simulink model "boost_and_two_level__1_sm_controller"  (R2021b)
settings: Solver=ode3  StartTime=0.0  StopTime=inf  FixedStep=2e-05  RelTol=1e-3
PostLoadFcn:
  | Boost_and_Two_Level_Inverter_param;
InitFcn:
  | Boost_and_Two_Level_Inverter_param;
undefined symbols (not defined in the file or in its folder): af15, arm1_g1, Boost2lvl_SFun, boost_I, boost_V, c62c8459, eHSx128_Gen4_Machines_IOConfig1, EX, fault_sw, Inv_PWM_Phases, Ts, v1, VC707_2, vin, vsrc1, vsrc2, vsrc3
libraries: opal_lib x5, rtio_opalrt_common x2, rtlab x1, ehsSchematicEditorSourceLib x1
PreSaveFcn:
  | try, efsUpdateVersionAnnotation, end
settings Model: ARTEMISmethode_block_infos=$$__separator__$$  Creator=PYRobert  LastModifiedBy=Grogu
settings SolverCC: AlgebraicLoopSolver=TrustRegion
settings DataIOCC: LimitDataPoints=on  SaveFormat=Array  SignalLoggingSaveFormat=ModelDataLogs  SaveOutput=off  SignalLogging=off  SaveTime=off  ReturnWorkspaceOutputs=off  SignalLoggingName=sigsOut
settings OptimizationCC: BlockReduction=off  OptimizeBlockIOStorage=off  BufferReuse=off  GlobalBufferReuse=off  ExpressionFolding=off  ExpressionDepthLimit=2147483647  LocalBlockOutputs=off  InitFltsAndDblsToZero=on  LifeSpan=inf  OptimizeDataStoreBuffers=off  BusAssignmentInplaceUpdate=off
settings DebuggingCC: SaveWithParameterizedLinksMsg=none  UnderspecifiedInitializationDetection=Classic  MergeDetectMultiDrivingBlocksExec=none  SignalResolutionControl=TryResolveAllWithWarning  InheritedTsInSrcMsg=none  MultiTaskDSMMsg=warning  MultiTaskCondExecSysMsg=none  ParameterOverflowMsg=none  FcnCallInpInsideContextMsg=warning  StateNameClashWarn=warning  SFUnexpectedBacktrackingDiag=warning  SFNoUnconditionalDefaultTransitionDiag=warning  SFExecutionAtInitializationDiag=none  SFMachineParentedDataDiag=warning  ArithmeticOperatorsInVariantConditions=warning
settings HardwareCC: ProdBitPerLong=64  ProdHWDeviceType=Intel->x86-64 (Linux 64)  TargetBitPerPointer=64  TargetBitPerSizeT=64  TargetBitPerPtrDiffT=64  TargetLongLongMode=on  TargetIntDivRoundTo=Zero  TargetEndianess=LittleEndian  TargetWordSize=64  TargetHWDeviceType=MATLAB Host  ProdEqTarget=off
settings ModelReferenceCC: PropagateSignalLabelsOutOfModel=off
settings SFSimCC: SimUseLocalCustomCode=off  CustomCodeUndefinedFunction=UseInterfaceOnly
settings RTWCC: GenCodeOnly=on  RTWUseLocalCustomCode=off
settings CodeAppCC: StateflowObjectComments=on
settings GRTTargetCC: TargetFcnLib=ansi_tfl_tmw.mat  TargetLangStandard=C89/C90 (ANSI)  CombineOutputUpdateFcns=off  GRTInterface=on
settings ConfigComp: CovMetricSettings=dw  CovSaveCumulativeToWorkspaceVar=on  CovSaveSingleToWorkspaceVar=on  CovExternalEMLEnable=off  CovSFcnEnable=off
settings SimscapeCC: SimscapeNormalizeSystem=off

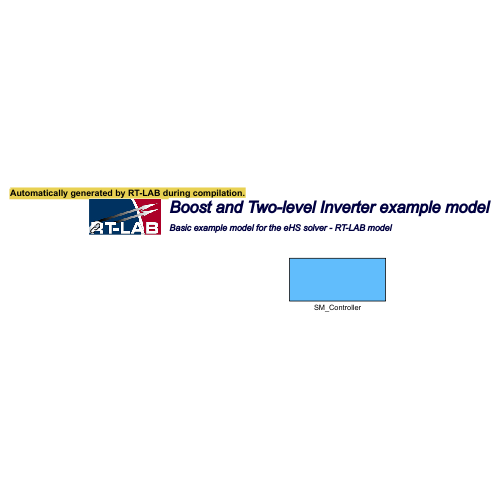
[thumbnail: Simulink's stored preview of the top-level diagram]
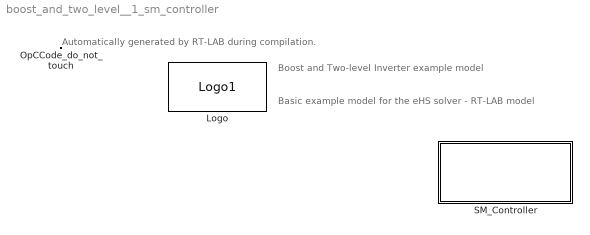
== system boost_and_two_level__1_sm_controller ==
  note: Boost and Two-level Inverter example model
  note: Basic example model for the eHS solver - RT-LAB model
  note: Automatically generated by RT-LAB during compilation.
  Logo : opal_lib/Logo1  vide=[]
  OpCCode_do_not_touch : opal_lib/Communication/OpCCode  SystemSampleTime=-1  VariantActivationTime=update diagram  Latency=0  AutoFrameSizeCalculation=off
  SM_Controller : Subsystem

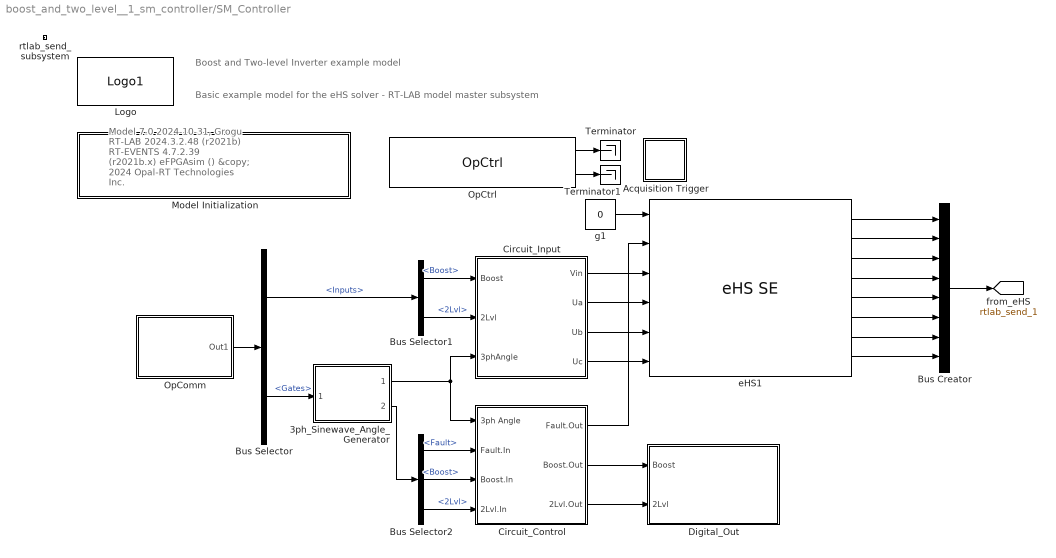
== system boost_and_two_level__1_sm_controller/SM_Controller ==
  note: Model 7.0 2024-10-31, Grogu
      | RT-LAB 2024.3.2.48 (r2021b)
      | RT-EVENTS 4.7.2.39 (r2021b.x)
      | eFPGAsim ()
      | &copy; 2024 Opal-RT Technologies Inc.
  note: Boost and Two-level Inverter example model
  note: Basic example model for the eHS solver - RT-LAB model master subsystem
  3ph_Sinewave_Angle_Generator : Subsystem
  Acquisition Trigger : Subsystem
  Bus Creator : BusCreator  Inputs=8
  Bus Selector : BusSelector  OutputSignals=Inputs,Gates
  Bus Selector1 : BusSelector  OutputSignals=Boost,2Lvl
  Bus Selector2 : BusSelector  OutputSignals=Fault,Boost,2Lvl
  Circuit_Control : Subsystem
  Circuit_Input : Subsystem
  Digital_Out : Subsystem
  Logo : opal_lib/Logo1  vide=[]
  Model Initialization : Subsystem  mask(Model Functions){InitFcnX=Boost_and_Two_Level_Inverter_param;, prel=off, posl=on, inif=on, strf=off}
      mask prompts: InitFcnX "Initialisation"; prel "Preload Function"; posl "PostLoad Function"; inif "InitFcn"; strf "StartFcn"
      mask init:
      | currentBlock = gcb;
      | root = bdroot(currentBlock);
      | 
      | if ~strcmp(get_param(root,'BlockDiagramType'),'library')
      |     if prel==1
      |         set_param(root, 'PreLoadFcn', InitFcnX);
      |     else
      |         set_param(root, 'PreLoadFcn', '');
      |     end
      |     if inif==1
      |         set_param(root, 'InitFcn', InitFcnX);
      |     else
      |         set_param(root, 'InitFcn', '');
      |     end
      |     if strf==1
      |         set_param(root, 'StartFcn', InitFcnX);
      |     else
      |         set_param(root, 'StartFcn', '');
      |     end
      |     if posl==1
      |         set_param(root, 'PostLoadFcn', InitFcnX);
      |     else
      |         set_param(root, 'PostLoadFcn', '');
      |     end
      | end
      | 
      | pos = get_param(currentBlock, 'Position');
      | width = pos(3) - pos(1); height = pos(4) - pos(2);
      | txt = [ upper(root) '\n' '- InitFcn. . . . . '  get_param(root, 'InitFcn') ];
      settings: CopyFcn=set_param(gcb,'LinkStatus','none')
      mask Display: text(5, height*0.5, txt, 'horizontalAlignment', 'left', 'verticalAlignment', 'middle') ;
  OpComm : Subsystem
      mask init:
      | opmaskdisplay('maskdisplay_block',gcb,'disp(''OpComm'')');
      mask Display:
      | patch([0 0.5 0.7 0],[1 1 0 0],[0.7 0.75 0.9]);
      | patch([1 0.53 0.73 1],[1 1 0 0],[1 0.8 0.7]);
      | plot([0 0 1 1 0],[0 1 1 0 0]);
      | disp('OpComm')
  OpCtrl : rtio_opalrt_common/OpCtrl  CtrlName='OpCtrl'  boardid=0  BitstreamFilename=VC707_2-EX-0001-3_6_0_818-eHSx128_Gen4_Machines_IOConfig1-35-61.bin  numconfig=-1  mode=Master  externalClock=off  decimRtsi=0  calibIO=off  SampleTime=0  loadinport=-1  BoardType=VC707  SecondaryPresent=off  sync_type=Audio  scope_enable=off  fsdFileName=VC707_2-EX-0001-3_4_0_820-eHSx128_Gen4_Machines_IOConfig1-35-4E.fsd  mismatch_disable=off
      settings: SourceProductName=RT-LAB I/O
  Terminator : Terminator
  Terminator1 : Terminator
  eHS1 : ehsSchematicEditorSourceLib/eHS SE  modelName=Boost2lvl_SFun - v1  modelUuid=c62c8459-3f79-48c0-af15-759a73c628dc  modelDisplayName=Boost2lvl_SFun  lastLoadedModelText=Circuit loaded on 09-Oct-2024 14:20:43  lastLoadedModelName=Boost2lvl_SFun - v1  lastLoadedModelUuid=c62c8459-3f79-48c0-af15-759a73c628dc  lastLoadedModelDisplayName=Boost2lvl_SFun - v1  triggerUpdate=on  timeStepInfo=Time Step: 230 ns (Min: 230 ns)  inputPins=arm1_g1,fault_sw,vin,vsrc1,vsrc2,vsrc3  outputPins=2Lvl_Ia,2Lvl_Ib,2Lvl_Ic,2Lvl_Va,2Lvl_Vb,2Lvl_Vc,boost_I,boost_V  loadPassed=1  firmwareName=VC707_2-EX-0001-3_6_0_818-eHSx128_Gen4_Machines_IOConfig1-35-61.bin  driverType=SFUN  ehsEffectiveLicense=x128  migrated=on  opCtrlName='OpCtrl'  autoConfigureFirmware=on  ehsFileName=Boost2lvl_SFun.ehs3  buildReportFile=C:\Working\git-repos\efpgasim-gitlab\efpgasim\Examples\Schematic_Editor_Workflow\eHS_Gen_4\Boost And Two Level Inverter\SFUN\Simulink\models\Boost_and_Two_Level_Inverter_Sfun\EFPGASIMConfig\logs\Boost2lvl_SFun\logs\eHSBuildReport.txt  displayBlockInfos=|
      | x128
      | Time Step: 230 ns (Min: 230 ns)
      settings: AttributesFormatString=%<opCtrlName>\n%<ehsFileName>\n%<displayBlockInfos>
  g1 : Constant  Value=0
  rtlab_send_subsystem : Subsystem  Priority=-100
      mask Display: text(0,0,'');
  tag scope: rtlab_send_1=global
  wires:
  OpComm/1(Out1) -> Bus Selector/1
  Circuit_Control/2(Boost.Out) -> Digital_Out/1(Boost)
  Circuit_Control/3(2Lvl.Out) -> Digital_Out/2(2Lvl)
  Bus Selector1/1 -> Circuit_Input/1(Boost)  "<Boost>"
  Bus Selector1/2 -> Circuit_Input/2(2Lvl)  "<2Lvl>"
  Bus Selector/1 -> Bus Selector1/1  "<Inputs>"
  Bus Selector/2 -> 3ph_Sinewave_Angle_Generator/1(Params.In)  "<Gates>"
  Bus Selector2/3 -> Circuit_Control/4(2Lvl.In)  "<2Lvl>"
  Bus Selector2/2 -> Circuit_Control/3(Boost.In)  "<Boost>"
  Bus Selector2/1 -> Circuit_Control/2(Fault.In)  "<Fault>"
  3ph_Sinewave_Angle_Generator/2(Params.Out) -> Bus Selector2/1
  3ph_Sinewave_Angle_Generator/1(3ph_Angle) -> Circuit_Input/3(3phAngle), Circuit_Control/1(3ph Angle)
  Bus Creator/1 -> [rtlab_send_1]
  Circuit_Control/1(Fault.Out) -> eHS1/2
  Circuit_Input/1(Vin) -> eHS1/3
  Circuit_Input/2(Ua) -> eHS1/4
  Circuit_Input/3(Ub) -> eHS1/5
  Circuit_Input/4(Uc) -> eHS1/6
  eHS1/2 -> Bus Creator/2
  eHS1/3 -> Bus Creator/3
  eHS1/4 -> Bus Creator/4
  eHS1/5 -> Bus Creator/5
  eHS1/6 -> Bus Creator/6
  eHS1/7 -> Bus Creator/7
  eHS1/8 -> Bus Creator/8
  g1/1 -> eHS1/1
  OpCtrl/1 -> Terminator/1
  OpCtrl/2 -> Terminator1/1
  eHS1/1 -> Bus Creator/1

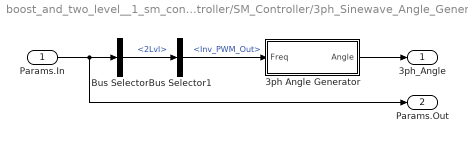
== system boost_and_two_level__1_sm_controller/SM_Controller/3ph_Sinewave_Angle_Generator ==
  Params.In : Inport
  3ph Angle Generator : Subsystem
  Bus Selector : BusSelector  OutputSignals=2Lvl
  Bus Selector1 : BusSelector  OutputSignals=Inv_PWM_Out
  3ph_Angle : Outport  VectorParamsAs1DForOutWhenUnconnected=off
  Params.Out : Outport  Port=2  VectorParamsAs1DForOutWhenUnconnected=off
  wires:
  Params.In/1 -> Params.Out/1, Bus Selector/1
  Bus Selector/1 -> Bus Selector1/1  "<2Lvl>"
  Bus Selector1/1 -> 3ph Angle Generator/1(Freq)  "<Inv_PWM_Out>"
  3ph Angle Generator/1(Angle) -> 3ph_Angle/1

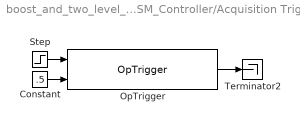
== system boost_and_two_level__1_sm_controller/SM_Controller/Acquisition Trigger ==
  Constant : Constant  Value=.5
  OpTrigger : rtlab/DataLogging/OpTrigger  Trig_Type=TRIGGER SIGNAL >= TRIGGER LEVEL  Trig_Offset=0  Acq_Group=1
      settings: SourceProductName=RT-LAB
  Step : Step  Time=0.5  SampleTime=Ts
  Terminator2 : Terminator
  wires:
  Constant/1 -> OpTrigger/2
  Step/1 -> OpTrigger/1
  OpTrigger/1 -> Terminator2/1

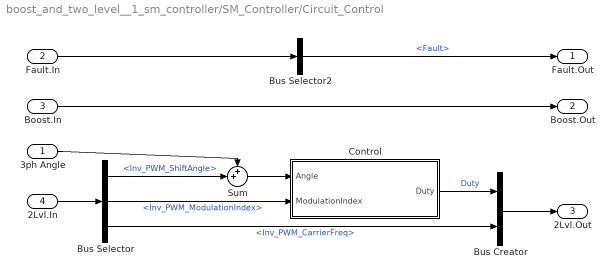
== system boost_and_two_level__1_sm_controller/SM_Controller/Circuit_Control ==
  3ph Angle : Inport
  Fault.In : Inport  Port=2
  Boost.In : Inport  Port=3
  2Lvl.In : Inport  Port=4
  Bus Creator : BusCreator  Inputs=2
  Bus Selector : BusSelector  OutputSignals=Inv_PWM_ShiftAngle,Inv_PWM_ModulationIndex,Inv_PWM_CarrierFreq
  Bus Selector2 : BusSelector  OutputSignals=Fault
  Control : Subsystem
  Sum : Sum  Inputs=++|
  Fault.Out : Outport  VectorParamsAs1DForOutWhenUnconnected=off
  Boost.Out : Outport  Port=2  VectorParamsAs1DForOutWhenUnconnected=off
  2Lvl.Out : Outport  Port=3  VectorParamsAs1DForOutWhenUnconnected=off
  wires:
  Boost.In/1 -> Boost.Out/1
  Bus Creator/1 -> 2Lvl.Out/1
  2Lvl.In/1 -> Bus Selector/1
  Fault.In/1 -> Bus Selector2/1
  Bus Selector2/1 -> Fault.Out/1  "<Fault>"
  Bus Selector/2 -> Control/2(ModulationIndex)  "<Inv_PWM_ModulationIndex>"
  Control/1(Duty) -> Bus Creator/1  "Duty"
  Bus Selector/3 -> Bus Creator/2  "<Inv_PWM_CarrierFreq>"
  Sum/1 -> Control/1(Angle)
  Bus Selector/1 -> Sum/2  "<Inv_PWM_ShiftAngle>"
  3ph Angle/1 -> Sum/1

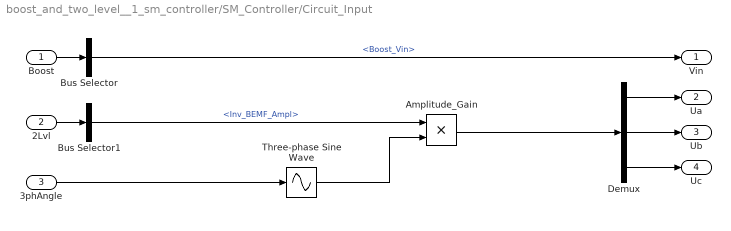
== system boost_and_two_level__1_sm_controller/SM_Controller/Circuit_Input ==
  Boost : Inport
  2Lvl : Inport  Port=2
  3phAngle : Inport  Port=3
  Amplitude_Gain : Product  RndMeth=Zero
  Bus Selector : BusSelector  OutputSignals=Boost_Vin
  Bus Selector1 : BusSelector  OutputSignals=Inv_BEMF_Ampl
  Demux : Demux  Outputs=3
  Three-phase Sine Wave : Sin  TimeSource=Use external signal  Phase=Inv_PWM_Phases
  Vin : Outport  VectorParamsAs1DForOutWhenUnconnected=off
  Ua : Outport  Port=2  VectorParamsAs1DForOutWhenUnconnected=off
  Ub : Outport  Port=3  VectorParamsAs1DForOutWhenUnconnected=off
  Uc : Outport  Port=4  VectorParamsAs1DForOutWhenUnconnected=off
  wires:
  Boost/1 -> Bus Selector/1
  Bus Selector/1 -> Vin/1  "<Boost_Vin>"
  2Lvl/1 -> Bus Selector1/1
  Demux/1 -> Ua/1
  Demux/2 -> Ub/1
  Demux/3 -> Uc/1
  Bus Selector1/1 -> Amplitude_Gain/1  "<Inv_BEMF_Ampl>"
  Amplitude_Gain/1 -> Demux/1
  Three-phase Sine Wave/1 -> Amplitude_Gain/2
  3phAngle/1 -> Three-phase Sine Wave/1

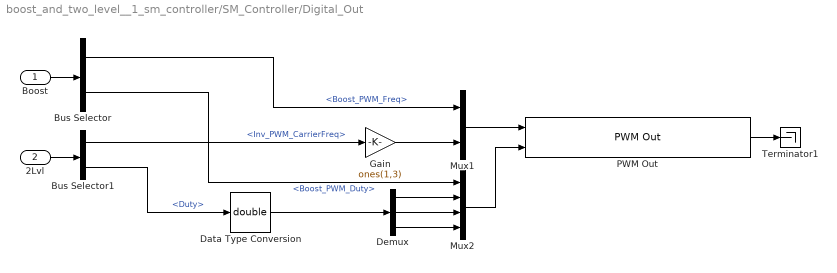
== system boost_and_two_level__1_sm_controller/SM_Controller/Digital_Out ==
  Boost : Inport
  2Lvl : Inport  Port=2
  Bus Selector : BusSelector  OutputSignals=Boost_PWM_Freq,Boost_PWM_Duty
  Bus Selector1 : BusSelector  OutputSignals=Inv_PWM_CarrierFreq,Duty
  Data Type Conversion : DataTypeConversion  OutDataTypeStr=double
  Demux : Demux  Outputs=3
  Gain : Gain  Gain=ones(1,3)
  Mux1 : Mux  Inputs=2
  Mux2 : Mux
  PWM Out : rtio_opalrt_common/PWM Out  CtrlName='OpCtrl'  portNb=11  FcnNos=Slot 2 Module B Subsection 1  size=64  maxcount=8  count=4  polarity=Active High  symMode=Asymmetric  rtPhaseDeadTimeEnabled=on  allowDisablingChannel=off  complementary=off  rtDeadTimeEnabled=off  deadTime=[0 0 0 0]  numchan=4  loadnb=4  rtPhaseShiftEnabled=off  initphase=[0 0 0 0]
      settings: AttributesFormatString=%<CtrlName>  SourceProductName=RT-LAB I/O
  Terminator1 : Terminator
  wires:
  Bus Selector/1 -> Mux1/1  "<Boost_PWM_Freq>"
  Bus Selector/2 -> Mux2/1  "<Boost_PWM_Duty>"
  Boost/1 -> Bus Selector/1
  2Lvl/1 -> Bus Selector1/1
  Bus Selector1/2 -> Data Type Conversion/1  "<Duty>"
  Data Type Conversion/1 -> Demux/1
  Bus Selector1/1 -> Gain/1  "<Inv_PWM_CarrierFreq>"
  Mux1/1 -> PWM Out/1
  Gain/1 -> Mux1/2
  Demux/2 -> Mux2/3
  Demux/1 -> Mux2/2
  Demux/3 -> Mux2/4
  Mux2/1 -> PWM Out/2
  PWM Out/1 -> Terminator1/1

== system boost_and_two_level__1_sm_controller/SM_Controller/Model Initialization ==

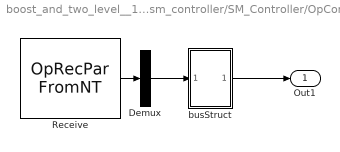
== system boost_and_two_level__1_sm_controller/SM_Controller/OpComm ==
  Demux : Demux  Outputs=[9]
  Receive : opal_lib/Communication/OpRecPar FromNT  Data_width=9  InitialConditions=[100;25;1;10000;0.7;55000;50;0.8;0.00349065850398866]
  busStruct : Subsystem
  Out1 : Outport
  wires:
  Demux/1 -> busStruct/1(In1)
  busStruct/1(Out1) -> Out1/1
  Receive/1 -> Demux/1

== system boost_and_two_level__1_sm_controller/SM_Controller/rtlab_send_subsystem ==
  Subsystem1 : Subsystem
  wires:
  [rtlab_send_1] -> Subsystem1/1(In1)

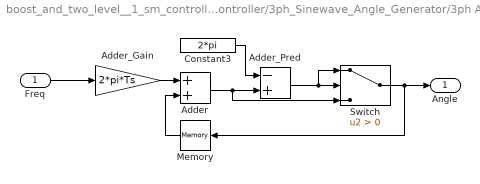
== system boost_and_two_level__1_sm_controller/SM_Controller/3ph_Sinewave_Angle_Generator/3ph Angle Generator ==
  Freq : Inport
  Adder : Sum
  Adder_Gain : Gain  Gain=2*pi*Ts  OutDataTypeStr=double
  Adder_Pred : Sum  Inputs=-+
  Constant3 : Constant  Value=2*pi  OutDataTypeStr=double
  Memory : Memory  InheritSampleTime=on
  Switch : Switch  Criteria=u2 > Threshold
  Angle : Outport  VectorParamsAs1DForOutWhenUnconnected=off
  wires:
  Memory/1 -> Adder/2
  Freq/1 -> Adder_Gain/1
  Adder/1 -> Switch/3, Adder_Pred/2
  Adder_Gain/1 -> Adder/1
  Constant3/1 -> Adder_Pred/1
  Switch/1 -> Angle/1, Memory/1
  Adder_Pred/1 -> Switch/2, Switch/1

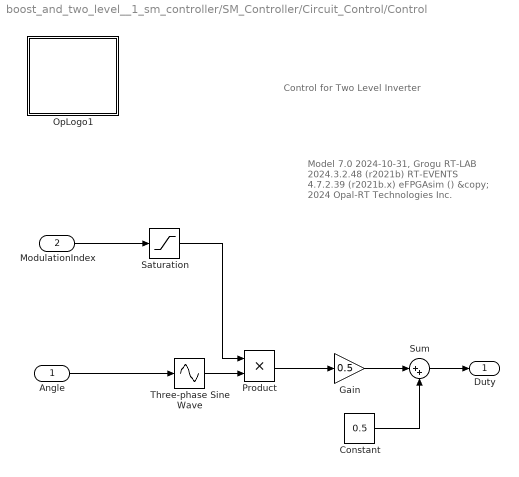
== system boost_and_two_level__1_sm_controller/SM_Controller/Circuit_Control/Control ==
  note: Control for Two Level Inverter
  note: Model 7.0 2024-10-31, Grogu
      | RT-LAB 2024.3.2.48 (r2021b)
      | RT-EVENTS 4.7.2.39 (r2021b.x)
      | eFPGAsim ()
      | &copy; 2024 Opal-RT Technologies Inc.
  Angle : Inport
  ModulationIndex : Inport  Port=2
  Constant : Constant  Value=0.5
  Gain : Gain  Gain=0.5
  OpLogo1 : Subsystem
  Product : Product  RndMeth=Zero
  Saturation : Saturate  UpperLimit=0.95  LowerLimit=0.05  OutDataTypeStr=Inherit: Inherit via back propagation
  Sum : Sum  Inputs=|++
  Three-phase Sine Wave : Sin  TimeSource=Use external signal  Phase=Inv_PWM_Phases
  Duty : Outport  VectorParamsAs1DForOutWhenUnconnected=off
  wires:
  ModulationIndex/1 -> Saturation/1
  Saturation/1 -> Product/1
  Product/1 -> Gain/1
  Gain/1 -> Sum/1
  Sum/1 -> Duty/1
  Constant/1 -> Sum/2
  Angle/1 -> Three-phase Sine Wave/1
  Three-phase Sine Wave/1 -> Product/2

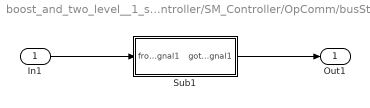
== system boost_and_two_level__1_sm_controller/SM_Controller/OpComm/busStruct ==
  In1 : Inport
  Sub1 : Subsystem
  Out1 : Outport
  wires:
  Sub1/1(goto_signal1) -> Out1/1
  In1/1 -> Sub1/1(from_signal1)

== system boost_and_two_level__1_sm_controller/SM_Controller/rtlab_send_subsystem/Subsystem1 ==
  In1 : Inport
  Mux : Mux  Inputs=1
  Send1 : opal_lib/Communication/OpSendToNT  Acqu_group=1
  wires:
  Mux/1 -> Send1/1
  In1/1 -> Mux/1

== system boost_and_two_level__1_sm_controller/SM_Controller/Circuit_Control/Control/OpLogo1 ==

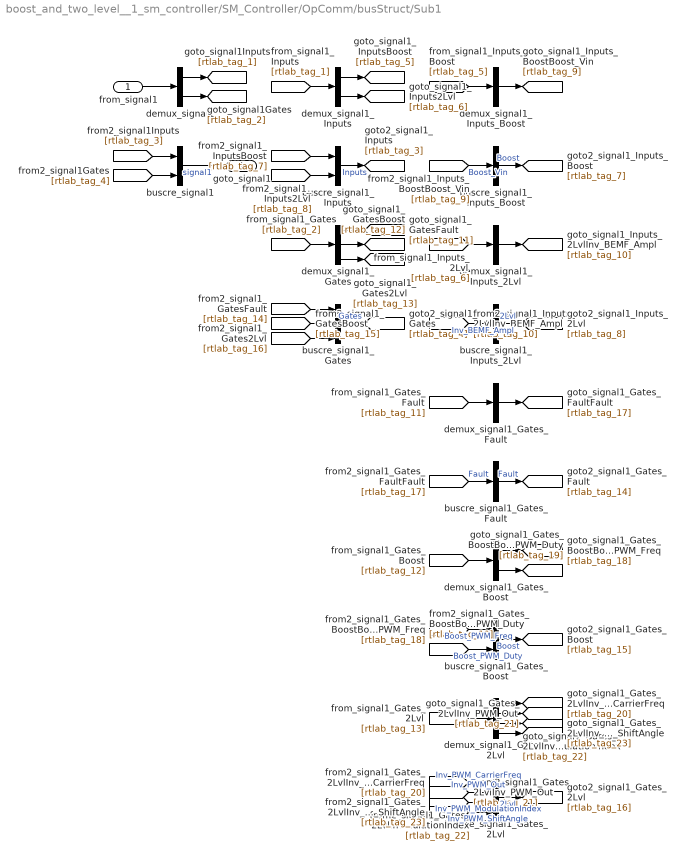
== system boost_and_two_level__1_sm_controller/SM_Controller/OpComm/busStruct/Sub1 ==
  from_signal1 : Inport
  buscre_signal1 : BusCreator  Inputs=2
  buscre_signal1_Gates : BusCreator  Inputs=3
  buscre_signal1_Gates_2Lvl : BusCreator  Inputs=4
  buscre_signal1_Gates_Boost : BusCreator  Inputs=2
  buscre_signal1_Gates_Fault : BusCreator  Inputs=1
  buscre_signal1_Inputs : BusCreator  Inputs=2
  buscre_signal1_Inputs_2Lvl : BusCreator  Inputs=1
  buscre_signal1_Inputs_Boost : BusCreator  Inputs=1
  demux_signal1 : Demux  Outputs="[2  7]"
  demux_signal1_Gates : Demux  Outputs="[1  2  4]"
  demux_signal1_Gates_2Lvl : Demux  Outputs="[1  1  1  1]"
  demux_signal1_Gates_Boost : Demux  Outputs="[1  1]"
  demux_signal1_Gates_Fault : Demux  Outputs=[1]
  demux_signal1_Inputs : Demux  Outputs="[1  1]"
  demux_signal1_Inputs_2Lvl : Demux  Outputs=[1]
  demux_signal1_Inputs_Boost : Demux  Outputs=[1]
  goto_signal1 : Outport
  wires:
  buscre_signal1_Gates_2Lvl/1 -> [rtlab_tag_16]  "2Lvl"
  [rtlab_tag_23] -> buscre_signal1_Gates_2Lvl/4  "Inv_PWM_ShiftAngle"
  [rtlab_tag_22] -> buscre_signal1_Gates_2Lvl/3  "Inv_PWM_ModulationIndex"
  [rtlab_tag_21] -> buscre_signal1_Gates_2Lvl/2  "Inv_PWM_Out"
  [rtlab_tag_20] -> buscre_signal1_Gates_2Lvl/1  "Inv_PWM_CarrierFreq"
  demux_signal1_Gates_2Lvl/4 -> [rtlab_tag_23]
  demux_signal1_Gates_2Lvl/3 -> [rtlab_tag_22]
  demux_signal1_Gates_2Lvl/2 -> [rtlab_tag_21]
  demux_signal1_Gates_2Lvl/1 -> [rtlab_tag_20]
  [rtlab_tag_13] -> demux_signal1_Gates_2Lvl/1
  buscre_signal1_Gates_Boost/1 -> [rtlab_tag_15]  "Boost"
  [rtlab_tag_19] -> buscre_signal1_Gates_Boost/2  "Boost_PWM_Duty"
  [rtlab_tag_18] -> buscre_signal1_Gates_Boost/1  "Boost_PWM_Freq"
  demux_signal1_Gates_Boost/2 -> [rtlab_tag_19]
  demux_signal1_Gates_Boost/1 -> [rtlab_tag_18]
  [rtlab_tag_12] -> demux_signal1_Gates_Boost/1
  buscre_signal1_Gates_Fault/1 -> [rtlab_tag_14]  "Fault"
  [rtlab_tag_17] -> buscre_signal1_Gates_Fault/1  "Fault"
  demux_signal1_Gates_Fault/1 -> [rtlab_tag_17]
  [rtlab_tag_11] -> demux_signal1_Gates_Fault/1
  buscre_signal1_Gates/1 -> [rtlab_tag_4]  "Gates"
  [rtlab_tag_16] -> buscre_signal1_Gates/3
  [rtlab_tag_15] -> buscre_signal1_Gates/2
  [rtlab_tag_14] -> buscre_signal1_Gates/1
  demux_signal1_Gates/3 -> [rtlab_tag_13]
  demux_signal1_Gates/2 -> [rtlab_tag_12]
  demux_signal1_Gates/1 -> [rtlab_tag_11]
  [rtlab_tag_2] -> demux_signal1_Gates/1
  buscre_signal1_Inputs_2Lvl/1 -> [rtlab_tag_8]  "2Lvl"
  [rtlab_tag_10] -> buscre_signal1_Inputs_2Lvl/1  "Inv_BEMF_Ampl"
  demux_signal1_Inputs_2Lvl/1 -> [rtlab_tag_10]
  [rtlab_tag_6] -> demux_signal1_Inputs_2Lvl/1
  buscre_signal1_Inputs_Boost/1 -> [rtlab_tag_7]  "Boost"
  [rtlab_tag_9] -> buscre_signal1_Inputs_Boost/1  "Boost_Vin"
  demux_signal1_Inputs_Boost/1 -> [rtlab_tag_9]
  [rtlab_tag_5] -> demux_signal1_Inputs_Boost/1
  buscre_signal1_Inputs/1 -> [rtlab_tag_3]  "Inputs"
  [rtlab_tag_8] -> buscre_signal1_Inputs/2
  [rtlab_tag_7] -> buscre_signal1_Inputs/1
  demux_signal1_Inputs/2 -> [rtlab_tag_6]
  demux_signal1_Inputs/1 -> [rtlab_tag_5]
  [rtlab_tag_1] -> demux_signal1_Inputs/1
  buscre_signal1/1 -> goto_signal1/1  "signal1"
  [rtlab_tag_4] -> buscre_signal1/2
  [rtlab_tag_3] -> buscre_signal1/1
  demux_signal1/2 -> [rtlab_tag_2]
  demux_signal1/1 -> [rtlab_tag_1]
  from_signal1/1 -> demux_signal1/1
